simulink model "DrivetrainHevP4_SSC"  (R2023b)
settings: Solver=ode23t  StartTime=0.0  StopTime=10.0  RelTol=1e-3
model workspace (MAT data in the model file):
  Aeff = 0.0314159265359
  Af = 2.27
  Apist_C0 = 0.0314159265359
  Apist_TCC = 0.001
  Bx = 10
  Cd = 0.25
  CoulFr_ShaftIn = 0
  Cx = 1.9
  DensAir = 1.293
  DerFac_C0 = 1
  DerFac_TCC = 1
  Drag_C0 = 0
  Drag_TCC = 0
  Dx = 1
  Eff_Diff = [0.98 0.98]
  Ex = 0.97
  FDrive = 3.32
  FDrive_P4 = 4.1
  FZMAX = 6570
  FZMIN = 0
  G = [0 1 2 3 4 5 6]
  G_o = 1
  Iyy = 0.8
  Iyy_Whl = 0.8
  JCa_Diff = 0.001
  JEng = 0.2
  JMot = 0.21
  JPl_Diff = 0.001
  JShIn = 1e-05
  JShOut = 0.15
  Jd = 0.025
  Ji = 0.21
  Jin_Cltch = 0.2
  Jout = [0.009 0.01 0.01 0.01 0.01 0.01 0.01]
  Jout_Cltch = 0.01
  Jt = 0.01
  Jw1 = 0.01
  Jw2 = 0.01
  K_c = 10000
  KinFr_C0 = 0.4
  KinFr_TCC = 0.3
  Lrel = 0.15
  Mass = 1623
  N = [0.001 4.212 2.637 1.8 1.386 1 0.772]
  NF = 2
  NR = 2
  N_P0 = 3
  Ndiff = 3.32
  Ndiff_P4 = 4.1
  Ndisk = 1
  Neff_C0 = 1
  Neff_TCC = 6
  PEng_C0 = 30000
  PEng_TCC = 100
  Pabs = 101325
  Press = 300000
  PwrThr_Diff = [0.001 0.001]
  RatFr_ShaftIn = 1.1
  Re = 0.327
  Reff = 0.11
  Reff_C0 = 0.11
  Reff_TCC = 130
  Rm = 0.15
  SprStff_ShaftIn = 10000
  StatFr_C0 = 0.45
  StatFr_TCC = 0.35
  T = 273
  Temp_bpts = [313 358]
  Trq_bpts = [25 50 75 100 150 200 250]
  UNLOADED_RADIUS = 0.336
  VXLOW = 2
  VisFr_Diff = [0.001 0.001]
  ViscFr_ShaftIn = 400
  aMy = 0.01
  a_CG = 1.09
  alphaMy = 0
  b = Simulink.Parameter
  b.Value = 400
  b.DataType = 'auto'
  b.Complexity = 'real'
  b.Dimensions = [1 1]
  bMy = 0
  b_CG = 1.7
  bd = 0.001
  betaMy = 1
  bi = 0.001
  bin_Cltch = 0.003
  bout = [0.003 0.003 0.003 0.003 0.003 0.003 0.003]
  bout_Cltch = 0.003
  br = 0.001
  bt = 0.001
  bw1 = 0.001
  bw2 = 0.001
  cGain = 100000
  cMy = 0
  disk_abore = 0.05
  domega_o = 0
  eta = [0.95 0.95 0.95 0.95 0.95 0.95 0.95]
  eta_diff = 0.98
  eta_tbl = [1 1 1 1 1 1 1 1 1 1 1 1 ... (1078 elements, 7x11x7x2)]
  g = 9.81
  h = 0.5
  k = Simulink.Parameter
  k.Value = 10000
  k.DataType = 'auto'
  k.Complexity = 'real'
  k.Dimensions = [1 1]
  kappamax = 1.5
  ki_c = 100000
  lam_x = 1
  mu_kinetic = 0.35
  mu_static = 0.45
  muk = 0.4
  mus = 0.45
  num_pads = 2
  omega_bpts = [500.383141081 749.619781963 1002.67614148 1250.9578527 1499.23956393 1747.52127515 1995.80298637 2501.9157054 2998.47912785 4001.15526933 5003.83141081]
  omega_c = Simulink.Parameter
  omega_c.Value = 500
  omega_c.DataType = 'auto'
  omega_c.Complexity = 'real'
  omega_c.Dimensions = [1 1]
  omega_o = 0
  omegai_o = 0
  omegal = 94.2477796077
  omegao = 0
  omegat_o = 0
  omegau = 83.7758040957
  omegaw1o = 0
  omegaw2o = 0
  p0 = 10000000
  phi = [0 0.5 0.6 0.7 0.8 0.87 0.92 0.94 0.96 0.97]
  phi_new = [0 0.5 0.6 0.7 0.8 0.87 0.92 0.94 0.96 0.97 0.99 1.02 1.1 1.2 1.3 1.4]
  philu = 0.85
  press = 700000
  psi = [12.2938 12.8588 13.1452 13.6285 14.6163 16.2675 19.3503 22.1046 29.9986 50]
  psi_new = [12.2938 12.8588 13.1452 13.6285 14.6163 16.2675 19.3503 22.1046 29.9986 50 48 41.76 34 30 29 29.5]
  tauC = 0.25
  tauTC = 0.1
  tau_s = 0.1
  theta_o = 0
  wc = 10
  win_o = 0
  wout_o = 0
  x_o = 0
  xdot_o = 0
  zeta = [2.232 1.5462 1.4058 1.2746 1.1528 1.0732 1.0192 0.9983 0.9983 0.9983]
  zeta_new = [2.232 1.5462 1.4058 1.2746 1.1528 1.0732 1.0192 0.9983 0.9983 0.9983 0.979797979798 1.04382929642 1.0320855615 1.01960784314 1.00904977376 1]
libraries: fl_lib x53, nesl_utility x34, sdl_lib x23, simulink x6, autolibpowerinfoutils x4
(part 1 of 3)
settings Model: DataDictionary=DrivetrainHevP4_SSC.sldd  EnableAccessToBaseWorkspace=off  ModifiedByFormat=The MathWorks, Inc.  Creator=The MathWorks, Inc.  LastModifiedBy=The MathWorks, Inc.
settings SolverCC: AlgebraicLoopSolver=TrustRegion  MaxZcPerStep=1
settings DebuggingCC: UnconnectedInputMsg=warning  UnconnectedOutputMsg=warning  UnconnectedLineMsg=warning  SubsystemReferenceDiagnosticForUnitTest=warning
settings ModelReferenceCC: EnableRefExpFcnMdlSchedulingChecks=on
settings RTWCC: DLArmComputeVersion=19.05

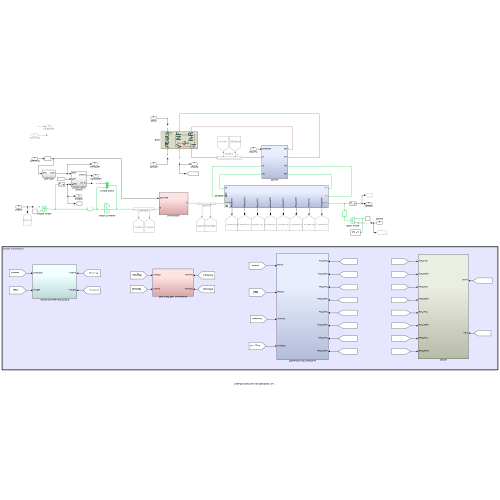
[thumbnail: Simulink's stored preview of the top-level diagram]
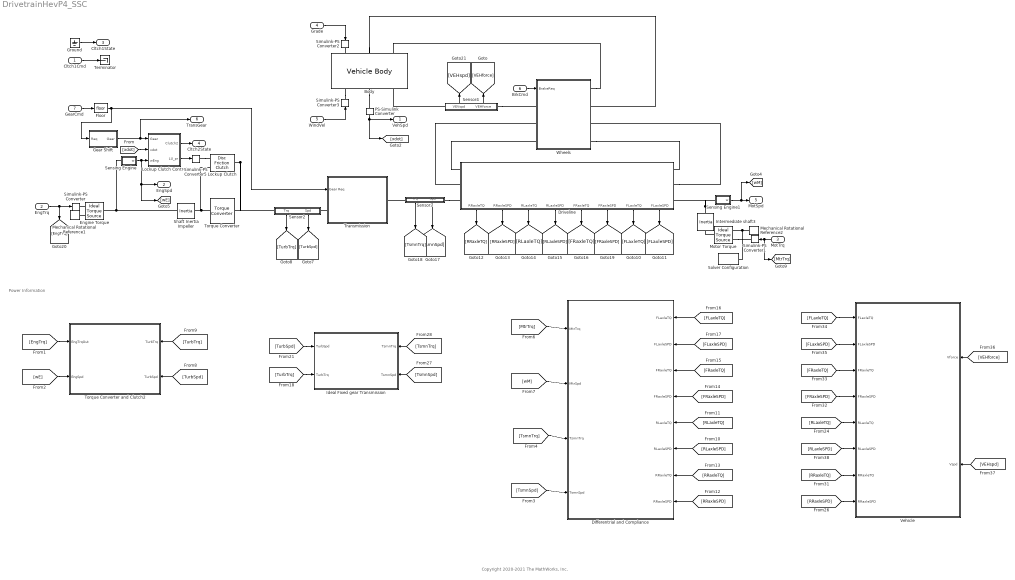
== system DrivetrainHevP4_SSC ==
  note: Power Information
  note: Copyright 2020-2021 The MathWorks, Inc.
  Cltch1Cmd : Inport
  EngTrq : Inport  Port=2
  MotTrq : Inport  Port=3
  Grade : Inport  Port=4  SampleTime=[-1, 0]
  WindVel : Inport  Port=5
  BrkCmd : Inport  Port=6
  GearCmd : Inport  Port=7
  Body : sdl_lib/Tires & Vehicles/Vehicle Body  mass=Mass kg  n_w=[NF NR]  x_f=a_CG m  x_r=b_CG m  y_c=h m  mass_var=simscape.enum.onoff.off  g=g m/s^2  liftoff_warning=simscape.enum.onoff.off  area=Af m^2  Cd=Cd  rho=DensAir kg/m^3  model_pitch=simscape.enum.onoff.off  inertia=4000 kg*m^2  suspension_model=sdl.enum.linearTLU.linear  k_f=1e4 N/m  b_f=1e4 N/(m/s)  k_r=1e4 N/m  b_r=1e4 N/(m/s)  k_f_TLU=[-2000, -1000, 0, 1000, 2000] N  x_f_TLU=[-.4, -.2, 0, .2, .4] m  b_f_TLU=[-200, -100, 0, 100, 200] N  v_f_TLU=[-4, -2, 0, 2, 4] m/s  k_r_TLU=[-2000, -1000, 0, 1000, 2000] N  x_r_TLU=[-.4, -.2, 0, .2, .4] m  b_r_TLU=[-200, -100, 0, 100, 200] N  v_r_TLU=[-4, -2, 0, 2, 4] m/s  interp_method=simscape.enum.interpolation.linear  extrap_method=simscape.enum.extrapolation.linear  model_hardstop=simscape.enum.onoff.off  upper_bound_f=.25 m  lower_bound_f=-.25 m  stop_k_f=1e6 N/m  stop_b_f=150 N/(m/s)  upper_bound_r=.25 m  lower_bound_r=-.25 m  stop_k_r=1e6 N/m  stop_b_r=150 N/(m/s)  initial_pitch=0 rad  initial_pitch_rate=0 rad/s  v_specify=on  v_priority=High  v=xdot_o m/s  v_nominal_specify=off  v_nominal_unit=m/s  v_nominal_value=1
  Differentrial and Compliance : Subsystem
      settings: PortSchema="{\"entries\":[{\"content\":{\"sides\":[{\"content\":{\"connectorIds\":[\"In1\",\"In2\",\"In3\",\"In4\",\"In5\",\"In6\",\"In7\",\"In8\"]},\"type\":\"ConnectorPlacement.EquallySpacedRectSide\",\"uuid\":\"bcf9a296-e69e-4ad9-a4a1-d979ea5df84c\"},{\"content\":{\"connectorIds\":[\"In9\",\"In10\",\"In11\",\"In12\"],\"side\":\"RIGHT\"},\"type\":\"ConnectorPlacement.EquallySpacedRectSide\",\"uuid\":\"3e14b290-259b-4f68-a20c-650572254037\"},{\"content\":{\"connectorIds\":[],\"side\":\"TOP\"},\"type\":\"ConnectorPlacement.EquallySpacedRectSide\",\"uuid\":\"59fe9e26-b0d5-4453-9443-e18838437669\"}]},\"type\":\"ConnectorPlacement.EquallySpacedConnector\",\"uuid\":\"2bd285bc-a7fd-4c69-a69e-79f070a662cd\"}],\"packageUris\":[\"http://schema.mathworks.com/mf0/Connector/R2020b\"],\"version\":\"1.0\"}"
  Driveline : Subsystem  Variant=on  VariantControlMode=label  VariantControl=Choice  LabelModeActiveChoice=2
      settings: PortSchema="{\"entries\":[{\"content\":{\"sides\":[{\"content\":{\"connectorIds\":[]},\"type\":\"ConnectorPlacement.EquallySpacedRectSide\",\"uuid\":\"1c8c165d-3f36-420a-b516-8f00de1791b0\"},{\"content\":{\"connectorIds\":[\"Out1\",\"Out2\",\"Out3\",\"Out4\",\"Out5\",\"Out6\",\"Out7\",\"Out8\"],\"side\":\"RIGHT\"},\"type\":\"ConnectorPlacement.EquallySpacedRectSide\",\"uuid\":\"7d84086b-e612-4967-bd32-18c88549edc3\"},{\"content\":{\"connectorIds\":[\"LConn1\",\"LConn2\",\"LConn3\"],\"side\":\"TOP\"},\"type\":\"ConnectorPlacement.EquallySpacedRectSide\",\"uuid\":\"03eded0d-6baf-42d1-b28a-0440e6f243a3\"},{\"content\":{\"connectorIds\":[\"RConn1\",\"RConn2\",\"RConn3\"],\"side\":\"BOTTOM\"},\"type\":\"ConnectorPlacement.EquallySpacedRectSide\",\"uuid\":\"6a626575-d497-4434-b7d6-b3b80bec74a2\"}]},\"type\":\"ConnectorPlacement.EquallySpacedConnector\",\"uuid\":\"aaae3d13-2aa2-4ebd-93dd-53292002797e\"}],\"packageUris\":[\"http://schema.mathworks.com/mf0/Connector/R2020b\"],\"version\":\"1.0\"}"
  Engine Torque : fl_lib/Mechanical/Mechanical Sources/Ideal Torque Source
  Floor : Rounding
  Gear Shift : Subsystem
  Ground : Ground
  Ideal Fixed gear Transmission : Subsystem
      settings: PortSchema="{\"entries\":[{\"content\":{\"sides\":[{\"content\":{\"connectorIds\":[\"In1\",\"In2\"]},\"type\":\"ConnectorPlacement.EquallySpacedRectSide\",\"uuid\":\"0efb6511-b0fb-4e7d-89a8-407c5ca1ba0b\"},{\"content\":{\"connectorIds\":[\"In3\",\"In4\"],\"side\":\"RIGHT\"},\"type\":\"ConnectorPlacement.EquallySpacedRectSide\",\"uuid\":\"d670609e-a10e-4a6b-a4e0-89dba182c718\"},{\"content\":{\"connectorIds\":[],\"side\":\"TOP\"},\"type\":\"ConnectorPlacement.EquallySpacedRectSide\",\"uuid\":\"605b7e6d-114c-4a56-8b24-1a2f6577cec3\"}]},\"type\":\"ConnectorPlacement.EquallySpacedConnector\",\"uuid\":\"2832aaad-a227-4ab8-9712-eb5d6f9fac3b\"}],\"packageUris\":[\"http://schema.mathworks.com/mf0/Connector/R2020b\"],\"version\":\"1.0\"}"
  Intermediate shaft3 : fl_lib/Mechanical/Rotational Elements/Inertia  inertia=JMot kg*m^2  num_ports=foundation.enum.numPorts2.two  w_specify=off  w_priority=High  w=0 rad/s  w_nominal_specify=off  w_nominal_unit=rad/s  w_nominal_value=1  t_specify=off  t_priority=High  t=0 N*m  t_nominal_specify=off  t_nominal_unit=N*m  t_nominal_value=1
      settings: InternalSimscapePortConfiguration="{\"Bottom\":[],\"Left\":[{\"id\":\"I\",\"label\":\"\",\"type\":\"foundation.mechanical.rotational.rotational\"}],\"Right\":[{\"id\":\"J\",\"label\":\"\",\"type\":\"foundation.mechanical.rotational.rotational\"}],\"Top\":[]}"
  Lockup Clutch : sdl_lib/Clutches/Disc Friction Clutch  geometry_model=sdl.enum.friction_geometry.radius  r_eff=Reff_TCC mm  d_o=150 mm  d_i=100 mm  nS=Neff_TCC  piston_area=Apist_TCC m^2  unidirectional=sdl.enum.directionality.bidirectional  friction_model=sdl.enum.friction_model_TLU_thermal.fixed  mu_w_vector=[0, 100, 1000] rad/s  temperature_TLU=[280, 300, 320] K  mu_static=StatFr_TCC  mu_static_vector=[.4, .38, .36]  mu_coulomb=KinFr_TCC  mu_coulomb_vector=[.3, .22, .19]  mu_coulomb_temp_vector=[.3, .28, .25]  mu_coulomb_matrix=[.34, .32, .3; .3, .28, .25; .25, .2, .15]  mu_interp_method=simscape.enum.interpolation.linear  mu_extrap_method=simscape.enum.extrapolation.linear  d_f=DerFac_TCC  w_tol=0.001 rad/s  pressure_min=PEng_TCC Pa  mu_visc=Drag_TCC N*m/(rad/s)  initial_state_locked=sdl.enum.initial_lock.unlocked  enable_faults=simscape.enum.onoff.off  fault_type=sdl.enum.clutchFault.lock  external_fault=simscape.enum.onoff.off  temporal_fault=simscape.enum.onoff.off  fault_time=5 s  report_fault=simscape.enum.assert.action.none  thermal_mass=25 kJ/K  T_init=300 K
      settings: InternalSimscapePortConfiguration="{\"Bottom\":[],\"Left\":[{\"id\":\"P\",\"label\":\"P\",\"type\":\"input\"},{\"id\":\"B\",\"label\":\"B\",\"type\":\"foundation.mechanical.rotational.rotational\"}],\"Right\":[{\"id\":\"F\",\"label\":\"F\",\"type\":\"foundation.mechanical.rotational.rotational\"}],\"Top\":[]}"
  Lockup Clutch Control : Subsystem
  Mechanical Rotational Reference1 : fl_lib/Mechanical/Rotational Elements/Mechanical Rotational Reference
  Mechanical Rotational Reference2 : fl_lib/Mechanical/Rotational Elements/Mechanical Rotational Reference
  Motor Torque : fl_lib/Mechanical/Mechanical Sources/Ideal Torque Source
  PS-Simulink Converter : nesl_utility/PS-Simulink Converter  PhysicalDomain=network_engine_domain  SubClassName=ps_output  LeftPortType=input  RightPortType=output  PseudoPeriodic=off  Frequencies=[]  VectorFormat=1-D array  Unit=m/s  AffineConversion=off
  Sensing Engine : Subsystem
  Sensing Engine1 : Subsystem
  Sensor2 : Subsystem
      settings: PortSchema="{\"entries\":[{\"content\":{\"sides\":[{\"content\":{\"connectorIds\":[\"LConn1\"]},\"type\":\"ConnectorPlacement.EquallySpacedRectSide\",\"uuid\":\"75ddaf40-3cfd-457e-a6d3-62b1cf2732a1\"},{\"content\":{\"connectorIds\":[\"RConn1\"],\"side\":\"RIGHT\"},\"type\":\"ConnectorPlacement.EquallySpacedRectSide\",\"uuid\":\"f96ccdb4-b20f-4a79-88cd-dc4740831283\"},{\"content\":{\"connectorIds\":[],\"side\":\"TOP\"},\"type\":\"ConnectorPlacement.EquallySpacedRectSide\",\"uuid\":\"7e11370f-51ad-4262-9bfc-30f014c3ad81\"},{\"content\":{\"connectorIds\":[\"Out1\",\"Out2\"],\"side\":\"BOTTOM\"},\"type\":\"ConnectorPlacement.EquallySpacedRectSide\",\"uuid\":\"80f49aed-f772-490c-9f60-3c9bebfa467a\"}]},\"type\":\"ConnectorPlacement.EquallySpacedConnector\",\"uuid\":\"e07fd8ac-10cb-405f-8306-46269df34852\"}],\"packageUris\":[\"http://schema.mathworks.com/mf0/Connector/R2020b\"],\"version\":\"1.0\"}"
  Sensor3 : Subsystem
      settings: PortSchema="{\"entries\":[{\"content\":{\"sides\":[{\"content\":{\"connectorIds\":[\"LConn1\"]},\"type\":\"ConnectorPlacement.EquallySpacedRectSide\",\"uuid\":\"49a89ebc-ab5d-4a78-a3cb-c5d68da1893f\"},{\"content\":{\"connectorIds\":[\"RConn1\"],\"side\":\"RIGHT\"},\"type\":\"ConnectorPlacement.EquallySpacedRectSide\",\"uuid\":\"2bd6ba44-e129-4b1c-b1af-ccb3382345fb\"},{\"content\":{\"connectorIds\":[],\"side\":\"TOP\"},\"type\":\"ConnectorPlacement.EquallySpacedRectSide\",\"uuid\":\"d8a8fe97-8b04-4dd9-b197-69b7723b7ab6\"},{\"content\":{\"connectorIds\":[\"Out1\",\"Out2\"],\"side\":\"BOTTOM\"},\"type\":\"ConnectorPlacement.EquallySpacedRectSide\",\"uuid\":\"49ab0c3f-5c19-4aba-9ae8-f8373bbb706f\"}]},\"type\":\"ConnectorPlacement.EquallySpacedConnector\",\"uuid\":\"f1c42ace-f3fa-47de-ae29-6a49b5c7e003\"}],\"packageUris\":[\"http://schema.mathworks.com/mf0/Connector/R2020b\"],\"version\":\"1.0\"}"
  Sensor4 : Subsystem
      settings: PortSchema="{\"entries\":[{\"content\":{\"sides\":[{\"content\":{\"connectorIds\":[\"LConn1\"]},\"type\":\"ConnectorPlacement.EquallySpacedRectSide\",\"uuid\":\"ac78708e-789e-4dda-b8fa-f180117c1afb\"},{\"content\":{\"connectorIds\":[\"RConn1\"],\"side\":\"RIGHT\"},\"type\":\"ConnectorPlacement.EquallySpacedRectSide\",\"uuid\":\"1aa3cffe-18fa-4015-b648-4424119ffd5e\"},{\"content\":{\"connectorIds\":[\"Out1\",\"Out2\"],\"side\":\"TOP\"},\"type\":\"ConnectorPlacement.EquallySpacedRectSide\",\"uuid\":\"48d6a6a5-2ce0-40f9-a78a-5bae6e2893e9\"},{\"content\":{\"connectorIds\":[],\"side\":\"BOTTOM\"},\"type\":\"ConnectorPlacement.EquallySpacedRectSide\",\"uuid\":\"bbbe6e0e-0439-464f-975b-cb5c5ae38f5b\"}]},\"type\":\"ConnectorPlacement.EquallySpacedConnector\",\"uuid\":\"45b4deed-0c42-43a0-aae3-55b4c8b471b5\"}],\"packageUris\":[\"http://schema.mathworks.com/mf0/Connector/R2020b\"],\"version\":\"1.0\"}"
  "Shaft Inertia Impeller " : fl_lib/Mechanical/Rotational Elements/Inertia  inertia=JEng kg*m^2  num_ports=foundation.enum.numPorts2.two  w_specify=off  w_priority=High  w=0 rad/s  w_nominal_specify=off  w_nominal_unit=rad/s  w_nominal_value=1  t_specify=off  t_priority=High  t=0 N*m  t_nominal_specify=off  t_nominal_unit=N*m  t_nominal_value=1
      settings: InternalSimscapePortConfiguration="{\"Bottom\":[],\"Left\":[{\"id\":\"I\",\"label\":\"\",\"type\":\"foundation.mechanical.rotational.rotational\"}],\"Right\":[{\"id\":\"J\",\"label\":\"\",\"type\":\"foundation.mechanical.rotational.rotational\"}],\"Top\":[]}"
  Simulink-PS Converter : nesl_utility/Simulink-PS Converter  PhysicalDomain=network_engine_domain  SubClassName=ps_input  LeftPortType=input  RightPortType=output  PseudoPeriodic=off  Frequencies=[]  NoiseDistribution=none  NoiseParameters=[]  Unit=N*m  AffineConversion=off  FilteringAndDerivatives=filter  SimscapeFilterOrder=1  InputFilterTimeConstant=0.01  UdotUserProvided=0
  Simulink-PS Converter1 : nesl_utility/Simulink-PS Converter  PhysicalDomain=network_engine_domain  SubClassName=ps_input  LeftPortType=input  RightPortType=output  PseudoPeriodic=off  Frequencies=[]  NoiseDistribution=none  NoiseParameters=[]  Unit=N*m  AffineConversion=off  FilteringAndDerivatives=filter  SimscapeFilterOrder=1  InputFilterTimeConstant=0.01  UdotUserProvided=0
  Simulink-PS Converter2 : nesl_utility/Simulink-PS Converter  PhysicalDomain=network_engine_domain  SubClassName=ps_input  LeftPortType=input  RightPortType=output  PseudoPeriodic=off  Frequencies=[]  NoiseDistribution=none  NoiseParameters=[]  Unit=deg  AffineConversion=off  FilteringAndDerivatives=provide  SimscapeFilterOrder=1  InputFilterTimeConstant=0.01  UdotUserProvided=0
  Simulink-PS Converter3 : nesl_utility/Simulink-PS Converter  PhysicalDomain=network_engine_domain  SubClassName=ps_input  LeftPortType=input  RightPortType=output  PseudoPeriodic=off  Frequencies=[]  NoiseDistribution=none  NoiseParameters=[]  Unit=m/s  AffineConversion=off  FilteringAndDerivatives=provide  SimscapeFilterOrder=1  InputFilterTimeConstant=0.01  UdotUserProvided=0
  Simulink-PS Converter5 : nesl_utility/Simulink-PS Converter  PhysicalDomain=network_engine_domain  SubClassName=ps_input  LeftPortType=input  RightPortType=output  PseudoPeriodic=off  Frequencies=[]  NoiseDistribution=none  NoiseParameters=[]  Unit=Pa  AffineConversion=off  FilteringAndDerivatives=filter  SimscapeFilterOrder=1  InputFilterTimeConstant=0.01  UdotUserProvided=0
  Solver Configuration : nesl_utility/Solver Configuration  PhysicalDomain=network_engine_domain  SubClassName=solver  LeftPortType=input  RightPortType=generic  Tones=[]  Harmonics=[]  SimulateNoise=off  Profile=off  UseLocalSampling=off  EnableSwitchedLinearOptims=on  FrequencyDomain=off  UseCCode=off  RelTol=0.001  AbsTol=1e-06  MinStep=1e-09  ToWorkspace=off  RevertToSquareIcSolve=off  NumHomotopyIterations=100  PhasorMode=off  PhasorModeNumHarmonics=1  ConsistencySolver=NEWTON_FTOL  IndexReductionMethod=DerivativeReplacement  DoDC=off  ResidualTolerance=1e-9  ConsistencyTolSource=GLOBAL  ConsistencyAbsTol=0.001  ConsistencyRelTol=0.001  ConsistencyTolFactor=0.001  UseLocalSolver=off  LocalSolverChoice=NE_BACKWARD_EULER_ADVANCER  ResolveIndetEquations=on  FunctionEvalNumThread=1  LocalSolverSampleTime=0.001  DoFixedCost=off  MaxNonlinIter=3  MaxModeIter=2  ComputeImpulses=off  ImpulseIterations=1  LinearAlgebra=Full  LinearAlgebraNumThread=0  EquationFormulation=NE_TIME_EF  DelaysMemoryBudget=1024  AutomaticFiltering=off  FilteringTimeConstant=0.001  PartitionStorageMethod=AS_NEEDED  PartitionMemoryBudget=1024  PartitionMethod=FAST  MultibodyUseLocalSolver=off  MultibodyLocalSolverChoice=ODE1  MultibodyLocalSolverSampleTime=0.001
  Terminator : Terminator
  Torque Converter : sdl_lib/Couplings & Drives/Torque Converter  coast_mode_modeling=sdl.enum.torqueConverterContinuousTwomode.continuous  SR_drive_tlu=[0, .5, .6, .7, .8, .87, .92, .94, .96, .97, 1]  TR_drive_tlu=[2.232, 1.5462, 1.4058, 1.2746, 1.1528, 1.0732, 1.0192, 1, 1, 1, 1]  CF_drive_tlu=1e-4 * [.72558, .66322, .63463, .59042, .51331, .4144, .29287, .22444, .12186, .04386, 0] m*N/rpm^2  SR_coast_tlu=[0, .5, .6, .7, .8, .87, .92, .94, .96, .97, 1]  CF_coast_tlu=1e-4 * [.5079, .4643, .4442, .4133, .3593, .2901, .205, .1571, .0853, .0307, 0] m*N/rpm^2  iniMode=sdl.enum.torqueConverterInitialMode.drive  delta_w=1 rpm  n_vector=phi  trq_vector=zeta  cf_vector_parameterization=sdl.enum.torqueConverterCFParameterization.SpeedToSqrtTorque  cf_vector_reference_speed=sdl.enum.torqueConverterCFReferenceSpeed.ImpellerSpeedLessThanOne  cf_vector=psi (rad/s)/(N*m)^0.5  cf_vector_sq=1e-3 * [6.616, 6.048, 5.787, 5.384, 4.681, 3.779, 2.671, 2.047, 1.111, .4] N*m/(rad/s)^2  interp_method=simscape.enum.interpolation.linear  extrap_method=simscape.enum.extrapolation.nearest  model_lag=sdl.enum.torqueConverterLagOnOff.LagOn  tau=tauTC s  initial_trq_ratio=0
      settings: InternalSimscapePortConfiguration="{\"Bottom\":[],\"Left\":[{\"id\":\"I\",\"label\":\"I\",\"type\":\"foundation.mechanical.rotational.rotational\"}],\"Right\":[{\"id\":\"T\",\"label\":\"T\",\"type\":\"foundation.mechanical.rotational.rotational\"}],\"Top\":[]}"
  Torque Converter and Clutch2 : Subsystem
      settings: PortSchema="{\"entries\":[{\"content\":{\"sides\":[{\"content\":{\"connectorIds\":[\"In1\",\"In2\"]},\"type\":\"ConnectorPlacement.EquallySpacedRectSide\",\"uuid\":\"b1f27cde-2e17-46f8-a7c4-32a68f2cd5d0\"},{\"content\":{\"connectorIds\":[\"In3\",\"In4\"],\"side\":\"RIGHT\"},\"type\":\"ConnectorPlacement.EquallySpacedRectSide\",\"uuid\":\"70f35508-9ee6-485d-898d-124f5b027daa\"},{\"content\":{\"connectorIds\":[],\"side\":\"TOP\"},\"type\":\"ConnectorPlacement.EquallySpacedRectSide\",\"uuid\":\"79e9d438-1519-46c3-8a92-70763141294d\"}]},\"type\":\"ConnectorPlacement.EquallySpacedConnector\",\"uuid\":\"bf0891ed-559f-4acc-9ae5-8e9e8cb9ba0c\"}],\"packageUris\":[\"http://schema.mathworks.com/mf0/Connector/R2020b\"],\"version\":\"1.0\"}"
  Transmission : Subsystem
  Vehicle : Subsystem
      settings: PortSchema="{\"entries\":[{\"content\":{\"sides\":[{\"content\":{\"connectorIds\":[\"In1\",\"In2\",\"In3\",\"In4\",\"In5\",\"In6\",\"In7\",\"In8\"]},\"type\":\"ConnectorPlacement.EquallySpacedRectSide\",\"uuid\":\"bcf9a296-e69e-4ad9-a4a1-d979ea5df84c\"},{\"content\":{\"connectorIds\":[\"In9\",\"In10\"],\"side\":\"RIGHT\"},\"type\":\"ConnectorPlacement.EquallySpacedRectSide\",\"uuid\":\"3e14b290-259b-4f68-a20c-650572254037\"},{\"content\":{\"connectorIds\":[],\"side\":\"TOP\"},\"type\":\"ConnectorPlacement.EquallySpacedRectSide\",\"uuid\":\"59fe9e26-b0d5-4453-9443-e18838437669\"}]},\"type\":\"ConnectorPlacement.EquallySpacedConnector\",\"uuid\":\"2bd285bc-a7fd-4c69-a69e-79f070a662cd\"}],\"packageUris\":[\"http://schema.mathworks.com/mf0/Connector/R2020b\"],\"version\":\"1.0\"}"
  Wheels : Subsystem
  VehSpd : Outport
  EngSpd : Outport  Port=2
  Cltch1State : Outport  Port=3
  Cltch2State : Outport  Port=4
  MotSpd : Outport  Port=5
  TransGear : Outport  Port=6  VectorParamsAs1DForOutWhenUnconnected=off  BusOutputAsStruct=on
  wires:
  GearCmd/1 -> Floor/1
  Ground/1 -> Cltch1State/1
  Gear Shift/1(Gear) -> TransGear/1, Lockup Clutch Control/1(Gear)
  [xdot] -> Lockup Clutch Control/2(xdot)
  Cltch1Cmd/1 -> Terminator/1
  Lockup Clutch Control/1(Clutch2) -> Cltch2State/1
  Floor/1 -> Transmission/1(Gear Req), Gear Shift/1(Req)
  Grade/1 -> Simulink-PS Converter2/1
  Sensing Engine/1(w) -> [wE], EngSpd/1, Lockup Clutch Control/3(wEng)
  PS-Simulink Converter/1 -> [xdot], VehSpd/1
  WindVel/1 -> Simulink-PS Converter3/1
  Sensing Engine1/1(w) -> [wM], MotSpd/1
  BrkCmd/1 -> Wheels/1(BrakeReq)
  EngTrq/1 -> Simulink-PS Converter/1, [EngTrq]
  MotTrq/1 -> [MtrTrq], Simulink-PS Converter1/1
  Lockup Clutch Control/2(LU_pr) -> Simulink-PS Converter5/1
  Sensor2/1(Trq) -> [TurbTrq]
  Sensor2/2(Spd) -> [TurbSpd]
  Sensor3/2(Spd) -> [TsmnSpd]
  Sensor3/1(Trq) -> [TsmnTrq]
  Driveline/1(RRaxleTQ) -> [RRaxleTQ]
  Driveline/2(RRaxleSPD) -> [RRaxleSPD]
  Driveline/3(RLaxleTQ) -> [RLaxleTQ]
  Driveline/4(RLaxleSPD) -> [RLaxleSPD]
  Driveline/5(FRaxleTQ) -> [FRaxleTQ]
  Driveline/6(FRaxleSPD) -> [FRaxleSPD]
  Driveline/7(FLaxleTQ) -> [FLaxleTQ]
  Driveline/8(FLaxleSPD) -> [FLaxleSPD]
  Sensor4/1(VEVspd) -> [VEHspd]
  Sensor4/2(VEHforce) -> [VEHforce]
  [wE] -> Torque Converter and Clutch2/2(EngSpd)
  [FLaxleSPD] -> Vehicle/2(FLaxleSPD)
  [RRaxleTQ] -> Differentrial and Compliance/2(RRaxleTQ)
  [RRaxleSPD] -> Vehicle/8(RRaxleSPD)
  [VEHforce] -> Vehicle/9(Vforce)
  [TurbTrq] -> Torque Converter and Clutch2/3(TurbTrq)
  [RLaxleSPD] -> Vehicle/6(RLaxleSPD)
  [FRaxleSPD] -> Vehicle/4(FRaxleSPD)
  [RLaxleSPD] -> Differentrial and Compliance/3(RLaxleSPD)
  [RRaxleTQ] -> Vehicle/7(RRaxleTQ)
  [RLaxleTQ] -> Differentrial and Compliance/4(RLaxleTQ)
  [FRaxleSPD] -> Differentrial and Compliance/5(FRaxleSPD)
  [RRaxleSPD] -> Differentrial and Compliance/1(RRaxleSPD)
  [VEHspd] -> Vehicle/10(Vspd)
  [FLaxleTQ] -> Vehicle/1(FLaxleTQ)
  [RLaxleTQ] -> Vehicle/5(RLaxleTQ)
  [EngTrq] -> Torque Converter and Clutch2/1(EngTrqOut)
  [MtrTrq] -> Differentrial and Compliance/12(MtrTrq)
  [FLaxleTQ] -> Differentrial and Compliance/8(FLaxleTQ)
  [FRaxleTQ] -> Vehicle/3(FRaxleTQ)
  [TurbTrq] -> Ideal Fixed gear Transmission/2(TurbTrq)
  [FRaxleTQ] -> Differentrial and Compliance/6(FRaxleTQ)
  [wM] -> Differentrial and Compliance/11(MtrSpd)
  [FLaxleSPD] -> Differentrial and Compliance/7(FLaxleSPD)
  [TsmnTrq] -> Differentrial and Compliance/10(TsmnTrq)
  [TurbSpd] -> Ideal Fixed gear Transmission/1(TurbSpd)
  [TsmnSpd] -> Differentrial and Compliance/9(TsmnSpd)
  [TsmnTrq] -> Ideal Fixed gear Transmission/3(TsmnTrq)
  [TurbSpd] -> Torque Converter and Clutch2/4(TurbSpd)
  [TsmnSpd] -> Ideal Fixed gear Transmission/4(TsmnSpd)
  connections:
  Mechanical Rotational Reference1/LConn1 -- Engine Torque/RConn2
  Body/RConn2 -- Wheels/RConn2
  Simulink-PS Converter5/RConn1 -- Lockup Clutch/LConn1
  Simulink-PS Converter/RConn1 -- Engine Torque/RConn1
  Body/LConn2 -- PS-Simulink Converter/LConn1
  Body/RConn3 -- Simulink-PS Converter2/RConn1
  Sensor3/LConn1 -- Transmission/RConn1
  Body/LConn3 -- Simulink-PS Converter3/RConn1
  Wheels/RConn1 -- Body/RConn1
  Motor Torque/RConn1 -- Simulink-PS Converter1/RConn1
  Mechanical Rotational Reference2/LConn1 -- Motor Torque/RConn2 -- Solver Configuration/RConn1
  Motor Torque/LConn1 -- Intermediate shaft3/LConn1
  Torque Converter/LConn1 -- Lockup Clutch/LConn2 -- "Shaft Inertia Impeller "/RConn1
  Sensor3/RConn1 -- Driveline/LConn3
  Driveline/RConn2 -- Wheels/RConn3
  Wheels/RConn4 -- Driveline/RConn1
  Sensing Engine/LConn1 -- "Shaft Inertia Impeller "/LConn1 -- Engine Torque/LConn1
  Intermediate shaft3/RConn1 -- Driveline/RConn3 -- Sensing Engine1/LConn1
  Lockup Clutch/RConn1 -- Sensor2/LConn1 -- Torque Converter/RConn1
  Transmission/LConn1 -- Sensor2/RConn1
  Wheels/LConn3 -- Driveline/LConn1
  Driveline/LConn2 -- Wheels/LConn2
  Sensor4/RConn1 -- Wheels/LConn1
  Sensor4/LConn1 -- Body/LConn1

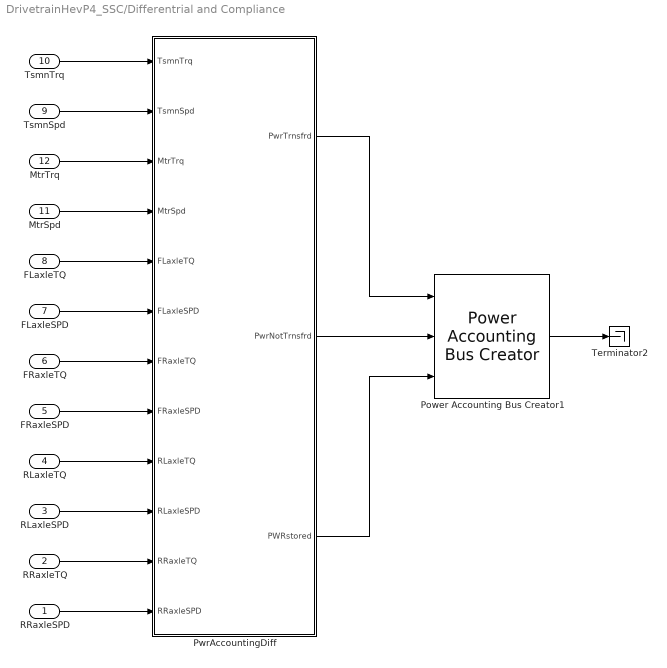
== system DrivetrainHevP4_SSC/Differentrial and Compliance ==
  RRaxleSPD : Inport
  RRaxleTQ : Inport  Port=2
  RLaxleSPD : Inport  Port=3
  RLaxleTQ : Inport  Port=4
  FRaxleSPD : Inport  Port=5
  FRaxleTQ : Inport  Port=6
  FLaxleSPD : Inport  Port=7
  FLaxleTQ : Inport  Port=8
  TsmnSpd : Inport  Port=9
  TsmnTrq : Inport  Port=10
  MtrSpd : Inport  Port=11
  MtrTrq : Inport  Port=12
  Power Accounting Bus Creator1 : autolibpowerinfoutils/Power Accounting Bus Creator  AssctBlkSelPopup=Parent  RefBlkName='diff'  PwrTrnsfrdCheckBox=on  PwrNotTrnsfrdCheckBox=on  PwrStoredCheckBox=on  aMode=aMode
  PwrAccountingDiff : Subsystem
  Terminator2 : Terminator
  wires:
  RLaxleTQ/1 -> PwrAccountingDiff/9(RLaxleTQ)
  RRaxleSPD/1 -> PwrAccountingDiff/12(RRaxleSPD)
  RLaxleSPD/1 -> PwrAccountingDiff/10(RLaxleSPD)
  FRaxleTQ/1 -> PwrAccountingDiff/7(FRaxleTQ)
  FLaxleTQ/1 -> PwrAccountingDiff/5(FLaxleTQ)
  FLaxleSPD/1 -> PwrAccountingDiff/6(FLaxleSPD)
  RRaxleTQ/1 -> PwrAccountingDiff/11(RRaxleTQ)
  TsmnTrq/1 -> PwrAccountingDiff/1(TsmnTrq)
  TsmnSpd/1 -> PwrAccountingDiff/2(TsmnSpd)
  PwrAccountingDiff/2(PwrNotTrnsfrd) -> Power Accounting Bus Creator1/2
  Power Accounting Bus Creator1/1 -> Terminator2/1
  PwrAccountingDiff/1(PwrTrnsfrd) -> Power Accounting Bus Creator1/1
  FRaxleSPD/1 -> PwrAccountingDiff/8(FRaxleSPD)
  PwrAccountingDiff/3(PWRstored) -> Power Accounting Bus Creator1/3
  MtrTrq/1 -> PwrAccountingDiff/3(MtrTrq)
  MtrSpd/1 -> PwrAccountingDiff/4(MtrSpd)

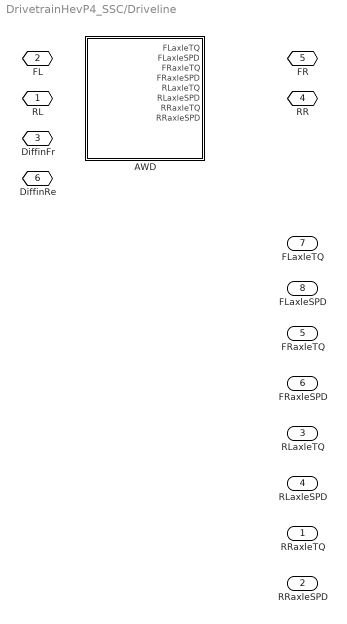
== system DrivetrainHevP4_SSC/Driveline ==
  AWD : Subsystem  VariantControl=2
  RL : PMIOPort  Side=Left
  FL : PMIOPort  Port=2  Side=Left
  DiffinFr : PMIOPort  Port=3  Side=Left
  RR : PMIOPort  Port=4  Side=Right
  FR : PMIOPort  Port=5  Side=Right
  DiffinRe : PMIOPort  Port=6  Side=Right
  RRaxleTQ : Outport
  RRaxleSPD : Outport  Port=2
  RLaxleTQ : Outport  Port=3
  RLaxleSPD : Outport  Port=4
  FRaxleTQ : Outport  Port=5
  FRaxleSPD : Outport  Port=6
  FLaxleTQ : Outport  Port=7
  FLaxleSPD : Outport  Port=8

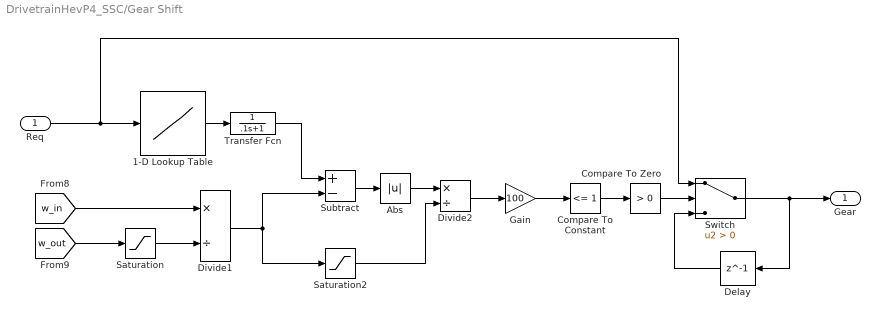
== system DrivetrainHevP4_SSC/Gear Shift ==
  Req : Inport
  1-D Lookup Table : Lookup_n-D  NumberOfTableDimensions=1  BreakpointsForDimension1=G  Table=N  InterpMethod=Flat  InternalRulePriority=Speed  OutDataTypeStr=Inherit: Inherit from 'Table data'  RndMeth=Simplest
  Abs : Abs  ZeroCross=off  SaturateOnIntegerOverflow=off
  Compare To Constant : simulink/Logic and Bit Operations/Compare To Constant  relop=<=  const=1  OutDataTypeStr=boolean  ZeroCross=off
  Compare To Zero : simulink/Logic and Bit Operations/Compare To Zero  relop=>  OutDataTypeStr=boolean
  Delay : Delay  DelayLength=1  InitialCondition=1
  Divide1 : Product  Inputs=*/
  Divide2 : Product  Inputs=*/
  Gain : Gain  Gain=100
  Saturation : Saturate  UpperLimit=inf  LowerLimit=1  ZeroCross=off
  Saturation2 : Saturate  UpperLimit=inf  LowerLimit=.1  ZeroCross=off
  Subtract : Sum  Inputs=+-
  Switch : Switch  Criteria=u2 > Threshold  SaturateOnIntegerOverflow=off  InputSameDT=off
  Transfer Fcn : TransferFcn  Denominator=[.1 1]
  Gear : Outport  VectorParamsAs1DForOutWhenUnconnected=off  BusOutputAsStruct=on
  wires:
  Divide1/1 -> Subtract/2, Saturation2/1
  Subtract/1 -> Abs/1
  Divide2/1 -> Gain/1
  Gain/1 -> Compare To Constant/1
  [w_out] -> Saturation/1
  [w_in] -> Divide1/1
  Abs/1 -> Divide2/1
  Req/1 -> Switch/1, 1-D Lookup Table/1
  1-D Lookup Table/1 -> Transfer Fcn/1
  Switch/1 -> Delay/1, Gear/1
  Compare To Zero/1 -> Switch/2
  Compare To Constant/1 -> Compare To Zero/1
  Delay/1 -> Switch/3
  Saturation/1 -> Divide1/2
  Transfer Fcn/1 -> Subtract/1
  Saturation2/1 -> Divide2/2

== system DrivetrainHevP4_SSC/Ideal Fixed gear Transmission ==
  TurbSpd : Inport
  TurbTrq : Inport  Port=2
  TsmnTrq : Inport  Port=3
  TsmnSpd : Inport  Port=4
  Power Accounting Bus Creator2 : autolibpowerinfoutils/Power Accounting Bus Creator  AssctBlkSelPopup=Parent  RefBlkName='diff'  PwrTrnsfrdCheckBox=on  PwrNotTrnsfrdCheckBox=on  PwrStoredCheckBox=on  aMode=aMode
  PwrAccountingDiff : Subsystem
  Terminator5 : Terminator
  wires:
  TurbTrq/1 -> PwrAccountingDiff/1(TurbTrq)
  TurbSpd/1 -> PwrAccountingDiff/2(TurbSpd)
  TsmnSpd/1 -> PwrAccountingDiff/4(TsmnSpd)
  TsmnTrq/1 -> PwrAccountingDiff/3(TsmnTrq)
  PwrAccountingDiff/3(PWRstored) -> Power Accounting Bus Creator2/3
  PwrAccountingDiff/1(PwrTrnsfrd) -> Power Accounting Bus Creator2/1
  PwrAccountingDiff/2(PwrNotTrnsfrd) -> Power Accounting Bus Creator2/2
  Power Accounting Bus Creator2/1 -> Terminator5/1

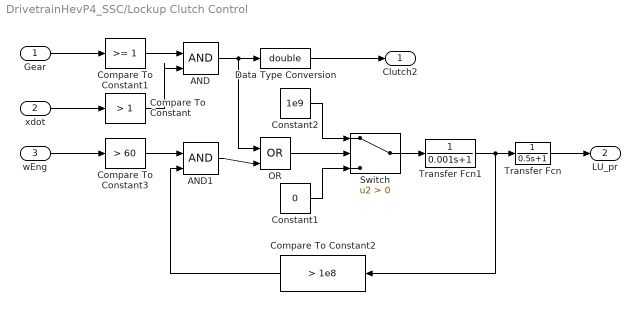
== system DrivetrainHevP4_SSC/Lockup Clutch Control ==
  Gear : Inport
  xdot : Inport  Port=2
  wEng : Inport  Port=3
  AND : Logic  IconShape=distinctive  AllPortsSameDT=off  OutDataTypeStr=boolean
  AND1 : Logic  IconShape=distinctive  AllPortsSameDT=off  OutDataTypeStr=boolean
  Compare To Constant : simulink/Logic and Bit Operations/Compare To Constant  relop=>  const=1  OutDataTypeStr=boolean  ZeroCross=off
  Compare To Constant1 : simulink/Logic and Bit Operations/Compare To Constant  relop=>=  const=1  OutDataTypeStr=boolean  ZeroCross=off
  Compare To Constant2 : simulink/Logic and Bit Operations/Compare To Constant  relop=>  const=1e8  OutDataTypeStr=boolean  ZeroCross=off
  Compare To Constant3 : simulink/Logic and Bit Operations/Compare To Constant  relop=>  const=60  OutDataTypeStr=boolean  ZeroCross=off
  Constant1 : Constant  Value=0
  Constant2 : Constant  Value=1e9
  Data Type Conversion : DataTypeConversion  OutDataTypeStr=double  SaturateOnIntegerOverflow=off  RndMeth=Floor
  OR : Logic  Operator=OR  IconShape=distinctive  AllPortsSameDT=off  OutDataTypeStr=boolean
  Switch : Switch  Criteria=u2 > Threshold  ZeroCross=off  SaturateOnIntegerOverflow=off  InputSameDT=off
  Transfer Fcn : TransferFcn  Denominator=[0.5 1]  ParameterTunability=Optimized
  Transfer Fcn1 : TransferFcn  Denominator=[0.001 1]
  Clutch2 : Outport  VectorParamsAs1DForOutWhenUnconnected=off
  LU_pr : Outport  Port=2  VectorParamsAs1DForOutWhenUnconnected=off
  wires:
  Transfer Fcn/1 -> LU_pr/1
  wEng/1 -> Compare To Constant3/1
  Transfer Fcn1/1 -> Compare To Constant2/1, Transfer Fcn/1
  Constant2/1 -> Switch/1
  Data Type Conversion/1 -> Clutch2/1
  Switch/1 -> Transfer Fcn1/1
  Gear/1 -> Compare To Constant1/1
  OR/1 -> Switch/2
  Compare To Constant2/1 -> AND1/2
  Compare To Constant3/1 -> AND1/1
  AND1/1 -> OR/2
  Constant1/1 -> Switch/3
  Compare To Constant1/1 -> AND/1
  Compare To Constant/1 -> AND/2
  AND/1 -> Data Type Conversion/1, OR/1
  xdot/1 -> Compare To Constant/1

== system DrivetrainHevP4_SSC/Sensing Engine ==
  Ideal Rotational Motion Sensor : fl_lib/Mechanical/Mechanical Sensors/Ideal Rotational Motion Sensor  reference=foundation.enum.MeasurementReference.difference  acceleration_port=false  velocity_port=true  position_port=true  wrap_angle=simscape.enum.onoff.off  offset=0 rev
  Mechanical Rotational Reference : fl_lib/Mechanical/Rotational Elements/Mechanical Rotational Reference
  PS Terminator : fl_lib/Physical Signals/Sinks/PS Terminator
  PS-Simulink Converter1 : nesl_utility/PS-Simulink Converter  PhysicalDomain=network_engine_domain  SubClassName=ps_output  LeftPortType=input  RightPortType=output  PseudoPeriodic=off  Frequencies=[]  VectorFormat=1-D array  Unit=rad/s  AffineConversion=off
  Saturation : Saturate  UpperLimit=inf  LowerLimit=eps  ZeroCross=off
  R : PMIOPort  Side=Left
  w : Outport
  wires:
  Saturation/1 -> w/1
  PS-Simulink Converter1/1 -> Saturation/1
  connections:
  Ideal Rotational Motion Sensor/RConn2 -- PS-Simulink Converter1/LConn1
  Ideal Rotational Motion Sensor/RConn1 -- Mechanical Rotational Reference/LConn1
  Ideal Rotational Motion Sensor/RConn3 -- PS Terminator/LConn1
  Ideal Rotational Motion Sensor/LConn1 -- R/RConn1

== system DrivetrainHevP4_SSC/Sensing Engine1 ==
  Ideal Rotational Motion Sensor : fl_lib/Mechanical/Mechanical Sensors/Ideal Rotational Motion Sensor  reference=foundation.enum.MeasurementReference.difference  acceleration_port=false  velocity_port=true  position_port=true  wrap_angle=simscape.enum.onoff.off  offset=0 rev
  Mechanical Rotational Reference : fl_lib/Mechanical/Rotational Elements/Mechanical Rotational Reference
  PS Terminator : fl_lib/Physical Signals/Sinks/PS Terminator
  PS-Simulink Converter1 : nesl_utility/PS-Simulink Converter  PhysicalDomain=network_engine_domain  SubClassName=ps_output  LeftPortType=input  RightPortType=output  PseudoPeriodic=off  Frequencies=[]  VectorFormat=1-D array  Unit=rad/s  AffineConversion=off
  Saturation : Saturate  UpperLimit=inf  LowerLimit=eps  ZeroCross=off
  R : PMIOPort  Side=Left
  w : Outport
  wires:
  PS-Simulink Converter1/1 -> Saturation/1
  Saturation/1 -> w/1
  connections:
  Ideal Rotational Motion Sensor/LConn1 -- R/RConn1
  Ideal Rotational Motion Sensor/RConn3 -- PS Terminator/LConn1
  Ideal Rotational Motion Sensor/RConn1 -- Mechanical Rotational Reference/LConn1
  Ideal Rotational Motion Sensor/RConn2 -- PS-Simulink Converter1/LConn1

== system DrivetrainHevP4_SSC/Sensor2 ==
  Ideal Rotational Motion Sensor1 : fl_lib/Mechanical/Mechanical Sensors/Ideal Rotational Motion Sensor  reference=foundation.enum.MeasurementReference.difference  acceleration_port=false  velocity_port=true  position_port=true  wrap_angle=simscape.enum.onoff.off  offset=0 rad
  Ideal Torque Sensor1 : fl_lib/Mechanical/Mechanical Sensors/Ideal Torque Sensor
  Mechanical Rotational Reference3 : fl_lib/Mechanical/Rotational Elements/Mechanical Rotational Reference
  PS Terminator1 : fl_lib/Physical Signals/Sinks/PS Terminator
  PS-Simulink Converter2 : nesl_utility/PS-Simulink Converter  PhysicalDomain=network_engine_domain  SubClassName=ps_output  LeftPortType=input  RightPortType=output  PseudoPeriodic=off  Frequencies=[]  VectorFormat=1-D array  Unit=inherit  AffineConversion=off
  PS-Simulink Converter3 : nesl_utility/PS-Simulink Converter  PhysicalDomain=network_engine_domain  SubClassName=ps_output  LeftPortType=input  RightPortType=output  PseudoPeriodic=off  Frequencies=[]  VectorFormat=1-D array  Unit=inherit  AffineConversion=off
  Saturation1 : Saturate  UpperLimit=inf  LowerLimit=eps  ZeroCross=off
  R : PMIOPort  Side=Left
  C : PMIOPort  Port=2  Side=Right
  Trq : Outport
  Spd : Outport  Port=2
  wires:
  PS-Simulink Converter2/1 -> Trq/1  "TurbTrq"
  PS-Simulink Converter3/1 -> Saturation1/1
  Saturation1/1 -> Spd/1  "TurbSpd"
  connections:
  Ideal Torque Sensor1/LConn1 -- R/RConn1 -- Ideal Rotational Motion Sensor1/LConn1
  PS-Simulink Converter2/LConn1 -- Ideal Torque Sensor1/RConn2
  Ideal Torque Sensor1/RConn1 -- C/RConn1
  PS-Simulink Converter3/LConn1 -- Ideal Rotational Motion Sensor1/RConn2
  PS Terminator1/LConn1 -- Ideal Rotational Motion Sensor1/RConn3
  Mechanical Rotational Reference3/LConn1 -- Ideal Rotational Motion Sensor1/RConn1

== system DrivetrainHevP4_SSC/Sensor3 ==
  DiffTQ : nesl_utility/PS-Simulink Converter  PhysicalDomain=network_engine_domain  SubClassName=ps_output  LeftPortType=input  RightPortType=output  PseudoPeriodic=off  Frequencies=[]  VectorFormat=1-D array  Unit=1  AffineConversion=off
  Ideal Rotational Motion Sensor : fl_lib/Mechanical/Mechanical Sensors/Ideal Rotational Motion Sensor  reference=foundation.enum.MeasurementReference.difference  acceleration_port=false  velocity_port=true  position_port=true  wrap_angle=simscape.enum.onoff.off  offset=0 rad
  Ideal Torque Sensor : fl_lib/Mechanical/Mechanical Sensors/Ideal Torque Sensor
  Mechanical Rotational Reference : fl_lib/Mechanical/Rotational Elements/Mechanical Rotational Reference
  PS Terminator : fl_lib/Physical Signals/Sinks/PS Terminator
  PS-Simulink Converter : nesl_utility/PS-Simulink Converter  PhysicalDomain=network_engine_domain  SubClassName=ps_output  LeftPortType=input  RightPortType=output  PseudoPeriodic=off  Frequencies=[]  VectorFormat=1-D array  Unit=inherit  AffineConversion=off
  R : PMIOPort  Side=Left
  C : PMIOPort  Port=2  Side=Right
  Trq : Outport
  Spd : Outport  Port=2
  wires:
  DiffTQ/1 -> Trq/1
  PS-Simulink Converter/1 -> Spd/1
  connections:
  DiffTQ/LConn1 -- Ideal Torque Sensor/RConn2
  Ideal Torque Sensor/RConn1 -- C/RConn1
  Ideal Torque Sensor/LConn1 -- R/RConn1 -- Ideal Rotational Motion Sensor/LConn1
  PS Terminator/LConn1 -- Ideal Rotational Motion Sensor/RConn3
  PS-Simulink Converter/LConn1 -- Ideal Rotational Motion Sensor/RConn2
  Mechanical Rotational Reference/LConn1 -- Ideal Rotational Motion Sensor/RConn1

== system DrivetrainHevP4_SSC/Sensor4 ==
  Force : nesl_utility/PS-Simulink Converter  PhysicalDomain=network_engine_domain  SubClassName=ps_output  LeftPortType=input  RightPortType=output  PseudoPeriodic=off  Frequencies=[]  VectorFormat=1-D array  Unit=1  AffineConversion=off
  Ideal Force Sensor : fl_lib/Mechanical/Mechanical Sensors/Ideal Force Sensor
  Ideal Translational Motion Sensor : fl_lib/Mechanical/Mechanical Sensors/Ideal Translational Motion Sensor  reference=foundation.enum.MeasurementReference.difference  acceleration_port=false  velocity_port=true  position_port=true  offset=0 m
  Mechanical Translational Reference : fl_lib/Mechanical/Translational Elements/Mechanical Translational Reference
  SPD : nesl_utility/PS-Simulink Converter  PhysicalDomain=network_engine_domain  SubClassName=ps_output  LeftPortType=input  RightPortType=output  PseudoPeriodic=off  Frequencies=[]  VectorFormat=1-D array  Unit=1  AffineConversion=off
  Out : PMIOPort  Side=Left
  H : PMIOPort  Port=2  Side=Right
  VEVspd : Outport
  VEHforce : Outport  Port=2
  wires:
  Force/1 -> VEHforce/1
  SPD/1 -> VEVspd/1
  connections:
  Ideal Force Sensor/RConn1 -- Out/RConn1
  Ideal Force Sensor/RConn2 -- Force/LConn1
  SPD/LConn1 -- Ideal Translational Motion Sensor/RConn2
  Ideal Force Sensor/LConn1 -- Ideal Translational Motion Sensor/LConn1 -- H/RConn1
  Mechanical Translational Reference/LConn1 -- Ideal Translational Motion Sensor/RConn1

== system DrivetrainHevP4_SSC/Torque Converter and Clutch2 ==
  EngTrqOut : Inport
  EngSpd : Inport  Port=2
  TurbTrq : Inport  Port=3
  TurbSpd : Inport  Port=4
  Power Accounting Bus Creator2 : autolibpowerinfoutils/Power Accounting Bus Creator  AssctBlkSelPopup=Parent  RefBlkName='diff'  PwrTrnsfrdCheckBox=on  PwrNotTrnsfrdCheckBox=on  PwrStoredCheckBox=on  aMode=aMode
  PwrAccountingDiff : Subsystem
  Terminator5 : Terminator
  wires:
  TurbTrq/1 -> PwrAccountingDiff/3(TurbTrq)
  TurbSpd/1 -> PwrAccountingDiff/4(TurbSpd)
  EngTrqOut/1 -> PwrAccountingDiff/2(EngTrqOut)
  PwrAccountingDiff/3(PWRstored) -> Power Accounting Bus Creator2/3
  PwrAccountingDiff/1(PwrTrnsfrd) -> Power Accounting Bus Creator2/1
  PwrAccountingDiff/2(PwrNotTrnsfrd) -> Power Accounting Bus Creator2/2
  Power Accounting Bus Creator2/1 -> Terminator5/1
  EngSpd/1 -> PwrAccountingDiff/1(EngSpd)
